simulink model "Hinf_simulation"  (R2018b)
settings: Solver=VariableStepAuto  StartTime=0.0  StopTime=25  FixedStep=1e-4  RelTol=1e-5
values from neighbouring files (symbols this model uses):
  Apass = [0, 1, 0, 0 ... (first row only)    [Vehicle_model_analysis.m]    (also in lab_3_model_uncertainity.m)
  Ask = [0 1 0 0 ... (first row only)    [Vehicle_model_analysis.m]    (also in genResponse2DOF_skyhook.m = [0, 1, 0, 0;-ks/ms, -T/ms, ks/ms, 0;0, 0, 0, 1;ks/mp, T/mp, ; getUpdatedModel.m; lab3_H_inf_ctrl.m; lab_3_model_uncertainity.m)
  Bpass = [0,0,0,0 ... (first row only)    [Vehicle_model_analysis.m]    (also in lab_3_model_uncertainity.m)
  Bsk = [0 0 0 0 ... (first row only)    [Vehicle_model_analysis.m]    (also in genResponse2DOF_skyhook.m = [0, 0; 0, 0; 0, 0; kp/mp, cp/mp]; getUpdatedModel.m; lab3_H_inf_ctrl.m; lab_3_model_uncertainity.m)
  Cpass = [0,1,0,0;0,0,0,1]    [Vehicle_model_analysis.m]    (also in lab_3_model_uncertainity.m = eye(4))
  Csk = [0 1 0 0 ... (first row only)    [Vehicle_model_analysis.m]    (also in genResponse2DOF_skyhook.m = [1, 0, 0, 0]; lab3_H_inf_ctrl.m; lab_3_model_uncertainity.m = eye(4))
  Dpass = zeros(2,4)    [Vehicle_model_analysis.m]    (also in lab_3_model_uncertainity.m = zeros(4,4))
  Dsk = zeros(2,4)    [Vehicle_model_analysis.m]    (also in genResponse2DOF_skyhook.m = [0,0]; lab3_H_inf_ctrl.m; lab_3_model_uncertainity.m = zeros(4,4))
undefined symbols (not defined in the file or in its folder): Ainf, Binf, Cinf, Dinf, sigbuilder_block
settings Model: Creator=Hp  LastModifiedBy=anirv
settings DataIOCC: ReturnWorkspaceOutputs=on

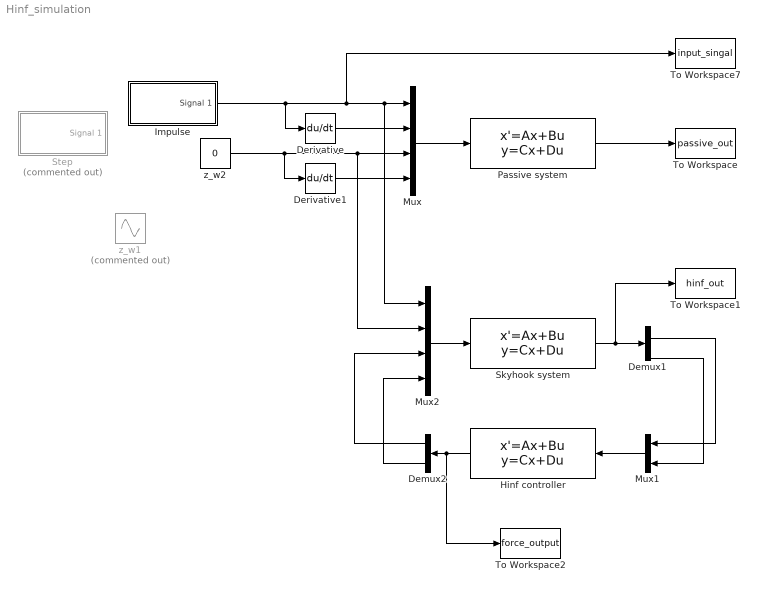
== system Hinf_simulation ==
  Demux1 : Demux
  Demux2 : Demux  Outputs=2
  Derivative : Derivative
  Derivative1 : Derivative
  Hinf controller : StateSpace  A=Ainf  B=Binf  C=Cinf  D=Dinf  InitialCondition=0
  Impulse : Subsystem  Tag=STV Subsys  LoadFcn=sigbuilder_block('load');  StartFcn=sigbuilder_block('start');  StopFcn=sigbuilder_block('stop');  ClipboardFcn=sigbuilder_block('clipboard');  mask(Sigbuilder block){tuvar=[0:10]}
      mask help: Simulink:masks:SigbuilderBlock_MD
      mask init:
      | if ~strcmp(get_param(bdroot(gcbh),'SimulationStatus'),'stopped') tuvar = sigbuilder_block('maskInit'); end
      settings: CopyFcn=sigbuilder_block('copy');  DeleteFcn=sigbuilder_block('delete');  ModelCloseFcn=sigbuilder_block('modelClose');  PreSaveFcn=sigbuilder_block('preSave');  PauseFcn=sigbuilder_block('pause');  ContinueFcn=sigbuilder_block('continue');  NameChangeFcn=sigbuilder_block('namechange');  OpenFcn=sigbuilder_block('open',[5.4 30 1141.2 522.6 ]);  CloseFcn=sigbuilder_block('close');
      mask Display: plot(0, 0, 100, 100,[2, 2, 32, 32, 2], [68, 8, 8, 68, 68],[32, 2], [38, 38], [32, 19, 2],[53, 60, 44], [32, 17, 17, 2],[16, 16, 31, 31]);txt = getActiveGroup(gcbh);text(2, 100, txt,'verticalAlignment', 'top');
  Mux : Mux
  Mux1 : Mux  Inputs=2
  Mux2 : Mux
  Passive system : StateSpace  A=Apass  B=Bpass  C=Cpass  D=Dpass  InitialCondition=0  ContinuousStateAttributes={'zs','zs_dot','chi','chi_dot'}
  Skyhook system : StateSpace  A=Ask  B=Bsk  C=Csk  D=Dsk  InitialCondition=0  ContinuousStateAttributes={'zs','zs_dot','chi','chi_dot'}
  Step : Subsystem  Tag=STV Subsys  Commented=on  LoadFcn=sigbuilder_block('load');  StartFcn=sigbuilder_block('start');  StopFcn=sigbuilder_block('stop');  ClipboardFcn=sigbuilder_block('clipboard');  mask(Sigbuilder block){tuvar=[0:10]}
      mask help: Simulink:masks:SigbuilderBlock_MD
      mask init:
      | if ~strcmp(get_param(bdroot(gcbh),'SimulationStatus'),'stopped') tuvar = sigbuilder_block('maskInit'); end
      settings: CopyFcn=sigbuilder_block('copy');  DeleteFcn=sigbuilder_block('delete');  ModelCloseFcn=sigbuilder_block('modelClose');  PreSaveFcn=sigbuilder_block('preSave');  PauseFcn=sigbuilder_block('pause');  ContinueFcn=sigbuilder_block('continue');  NameChangeFcn=sigbuilder_block('namechange');  OpenFcn=sigbuilder_block('open',[-1023 34.8 949.2 474.6 ]);  CloseFcn=sigbuilder_block('close');
      mask Display: plot(0, 0, 100, 100,[2, 2, 32, 32, 2], [68, 8, 8, 68, 68],[32, 2], [38, 38], [32, 19, 2],[53, 60, 44], [32, 17, 17, 2],[16, 16, 31, 31]);txt = getActiveGroup(gcbh);text(2, 100, txt,'verticalAlignment', 'top');
  To Workspace : ToWorkspace  VariableName=passive_out  SaveFormat=Timeseries  SampleTime=-1
  To Workspace1 : ToWorkspace  VariableName=hinf_out  SaveFormat=Timeseries  SampleTime=-1
  To Workspace2 : ToWorkspace  VariableName=force_output  SaveFormat=Timeseries  SampleTime=-1
  To Workspace7 : ToWorkspace  VariableName=input_singal  SaveFormat=Timeseries  SampleTime=-1
  z_w1 : Sin  Commented=on  Amplitude=0.01  Frequency=6.28  SampleTime=0
  z_w2 : Constant  Value=0
  wires:
  Derivative/1 -> Mux/2
  Mux/1 -> Passive system/1
  Impulse/1(Signal 1) -> Derivative/1, To Workspace7/1, Mux/1, Mux2/1
  z_w2/1 -> Derivative1/1, Mux/3, Mux2/2
  Derivative1/1 -> Mux/4
  Passive system/1 -> To Workspace/1
  Skyhook system/1 -> To Workspace1/1, Demux1/1
  Mux2/1 -> Skyhook system/1
  Hinf controller/1 -> To Workspace2/1, Demux2/1
  Demux2/1 -> Mux2/3
  Demux2/2 -> Mux2/4
  Demux1/2 -> Mux1/1
  Demux1/4 -> Mux1/2
  Mux1/1 -> Hinf controller/1

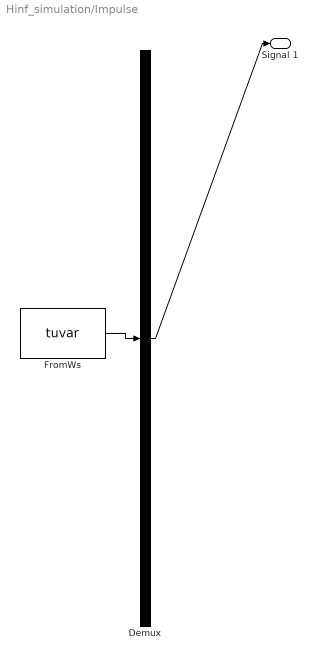
== system Hinf_simulation/Impulse ==
  Demux : Demux  Tag=STV Demux  Outputs=1
  FromWs : FromWorkspace  Tag=STV FromWs  VariableName=tuvar  SampleTime=0
      SigBuilderData=|
      | common.afterFinalStr = 'Extrapolate'
      | common.sampleTime = 0
      | dataSet.timeRange = [0 60]
      | dataSet.name = 'Group 1'
      | sbobj.Groups.Name = 'Group 1'
      | sbobj.Groups.Signals.Name = 'Signal 1'
      | sbobj.Groups.Signals.XData = [0 9.995 9.995 10.005 10.005 60]
      | sbobj.Groups.Signals.YData = [0 0 0.03 0.03 0 0]
      | sbobj.Groups.TimeRange = [0 60]
  Signal 1 : Outport  Tag=STV Outport
  wires:
  FromWs/1 -> Demux/1
  Demux/1 -> Signal 1/1

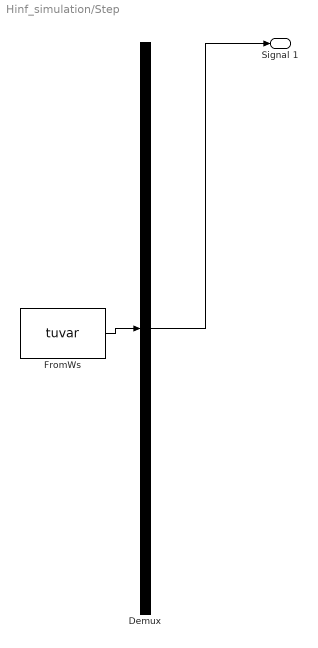
== system Hinf_simulation/Step ==
  Demux : Demux  Tag=STV Demux  Outputs=1
  FromWs : FromWorkspace  Tag=STV FromWs  VariableName=tuvar  SampleTime=0
      SigBuilderData=|
      | common.afterFinalStr = 'Extrapolate'
      | common.sampleTime = 0
      | dataSet.timeRange = [0 60]
      | dataSet.name = 'Group 1'
      | sbobj.Groups.Name = 'Group 1'
      | sbobj.Groups.Signals.Name = 'Signal 1'
      | sbobj.Groups.Signals.XData = [0 33.3 33.3 60]
      | sbobj.Groups.Signals.YData = [0.03 0.03 0 0]
      | sbobj.Groups.TimeRange = [0 60]
  Signal 1 : Outport  Tag=STV Outport  VectorParamsAs1DForOutWhenUnconnected=on
  wires:
  Demux/1 -> Signal 1/1
  FromWs/1 -> Demux/1
